simulink model "TS3"  (R2024b)
settings: Solver=VariableStepAuto  StartTime=0.0  StopTime=10  RelTol=1e-3
values from neighbouring files (symbols this model uses):
  k1 = 0.08    [tema1.m]    (also in tema3.m = 1)
  k2 = 0.5    [tema3.m]
  k3 = -0.5    [tema3.m]
  k4 = 1.40    (= 1.4)    [tema3.m]
  k5 = 1.65    [tema3.m]
  k6 = 2    [tema3.m]
settings Model: Creator=albertrosca  LastModifiedBy=albertrosca

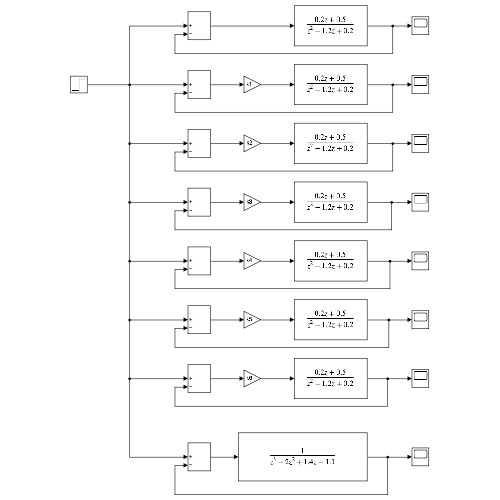
[thumbnail: Simulink's stored preview of the top-level diagram]
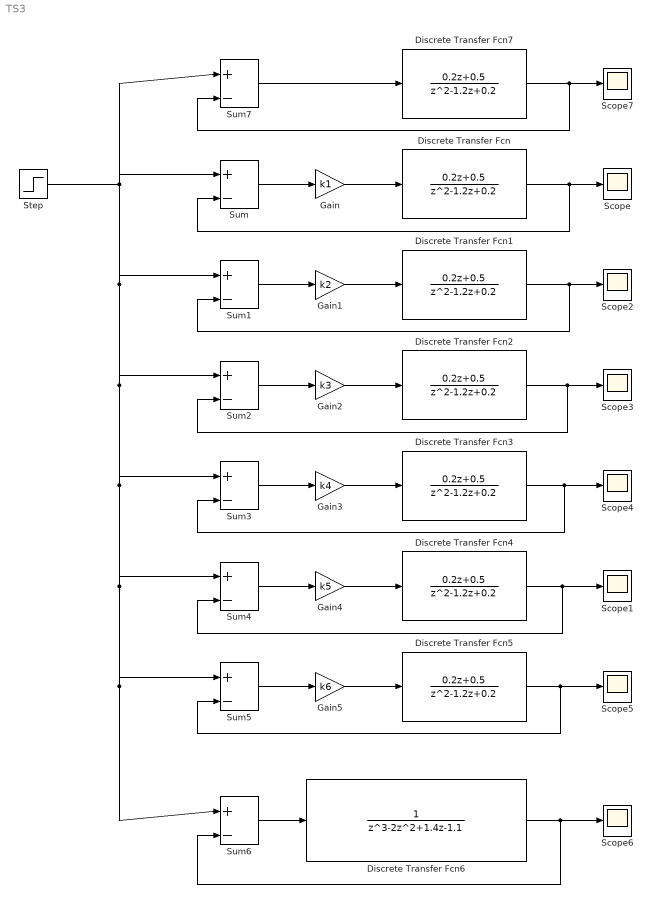
== system TS3 ==
  Discrete Transfer Fcn{,1..5,7} (7 alike) : DiscreteTransferFcn  Numerator=[0.2 0.5]  Denominator=[1 -1.2 0.2]  SampleTime=0.005
  Discrete Transfer Fcn6 : DiscreteTransferFcn  Numerator=[ 1 ]  Denominator=[ 1 -2 1.4 -1.1 ]  SampleTime=0.005
  Gain : Gain  Gain=k1
  Gain1 : Gain  Gain=k2
  Gain2 : Gain  Gain=k3
  Gain3 : Gain  Gain=k4
  Gain4 : Gain  Gain=k5
  Gain5 : Gain  Gain=k6
  Scope{,1..7} (8 alike) : Scope
  Step : Step  Time=0  SampleTime=0.1
  Sum{,1..7} (8 alike) : Sum  Inputs=|+-
  wires:
  Sum/1 -> Gain/1
  Sum1/1 -> Gain1/1
  Sum2/1 -> Gain2/1
  Sum3/1 -> Gain3/1
  Sum4/1 -> Gain4/1
  Sum5/1 -> Gain5/1
  Discrete Transfer Fcn/1 -> Scope/1, Sum/2
  Discrete Transfer Fcn1/1 -> Scope2/1, Sum1/2
  Discrete Transfer Fcn2/1 -> Scope3/1, Sum2/2
  Discrete Transfer Fcn3/1 -> Scope4/1, Sum3/2
  Discrete Transfer Fcn4/1 -> Scope1/1, Sum4/2
  Discrete Transfer Fcn5/1 -> Scope5/1, Sum5/2
  Gain/1 -> Discrete Transfer Fcn/1
  Gain3/1 -> Discrete Transfer Fcn3/1
  Gain4/1 -> Discrete Transfer Fcn4/1
  Gain5/1 -> Discrete Transfer Fcn5/1
  Gain1/1 -> Discrete Transfer Fcn1/1
  Gain2/1 -> Discrete Transfer Fcn2/1
  Sum6/1 -> Discrete Transfer Fcn6/1
  Discrete Transfer Fcn6/1 -> Scope6/1, Sum6/2
  Discrete Transfer Fcn7/1 -> Scope7/1, Sum7/2
  Sum7/1 -> Discrete Transfer Fcn7/1
  Step/1 -> Sum7/1, Sum/1, Sum6/1, Sum5/1, Sum4/1, Sum3/1, Sum2/1, Sum1/1
